simulink model "Copter_Plane_V10_sim_jy"  (R2021a)
settings: Solver=ode1  StartTime=0.0  StopTime=200  FixedStep=dt  RelTol=1e-3
undefined symbols (not defined in the file or in its folder): AC_Attitude, AC_PosControl, algo_accel_target_0, algo_accel_target_1, algo_accel_target_2, algo_arspeed, algo_attitude_target_euler_angle_0, algo_attitude_target_euler_angle_1, algo_attitude_target_euler_angle_2, algo_attitude_target_euler_rate_0, algo_attitude_target_euler_rate_1, algo_attitude_target_euler_rate_2, algo_climb_rate_cms, algo_curPathPoint_LLA_0, algo_curPathPoint_LLA_1, algo_curPosNED_0, algo_curPosNED_1, algo_curr_alt, algo_curr_pos_0, algo_curr_pos_1, algo_curr_vel_0, algo_curr_vel_1, algo_curr_vel_2, algo_current_loc_0, algo_current_loc_1, algo_curVelNED_0, algo_curVelNED_1, algo_flightControlMode, algo_flightTaskMode, algo_heightCmd_sl, algo_hgt_dem, algo_k_aileron, algo_k_elevator, algo_k_rudder, algo_k_throttle, algo_latAccDem, algo_limit_pos_up, algo_maxClimbSpeed, algo_mode, algo_nav_pitch_cd, algo_nav_roll, algo_pitch, algo_pitch_dem, algo_pitch_in, algo_pitch_target_pilot, algo_plane_mode, algo_pos_target_0, algo_pos_target_1, algo_pos_target_2, algo_prePathPoint_LLA_0, algo_prePathPoint_LLA_1, algo_pwm_out_1, algo_pwm_out_2, algo_pwm_out_3, algo_pwm_out_4, algo_rate_target_ang_vel_0, algo_rate_target_ang_vel_1, algo_rate_target_ang_vel_2, algo_remote_ct_st_pitch, algo_remote_ct_st_roll ... (+39)
libraries: aerolibasang x1, sharedtransform x1
(part 2 of 2)

== matlab function Copter_Plane_V10_sim_jy/input_euler_angle_roll_pitch_euler_rate_yaw ==
  data: GRAVITY_MSS data_store_memory; HD data_store_memory; dt data_store_memory; LOCATION_SCALING_FACTOR_INV data_store_memory; PathModeOut_sl data_store_memory; plane_mode data_store_memory; algo_remote_ct_st data_store_memory; algo_dbg_param data_store_memory; Curr_sate data_store_memory; systime data_store_memory; Test_w data_store_memory; AC_rate_pitch_pid data_store_memory; AC_rate_roll_pid data_store_memory; AC_rate_yaw_pid data_store_memory; AC_PosControl data_store_memory; AP_rate_roll data_store_memory; AP_rate_pitch data_store_memory; AP_rate_yaw data_store_memory; AP_TECS data_store_memory; AP_L1 data_store_memory; Plane data_store_memory; SRV_Channel data_store_memory; AC_Attitude data_store_memory; AP_Motors data_store_memory; Copter_Plane data_store_memory; LOCATION_SCALING_FACTOR data_store_memory; SINS data_store_memory; SlewLimiter data_store_memory
function copter_plane_run

run_remote();
load_Curr_sate();
loc_run();
load_inint();
sin_step_test();
%%%%%%%%%%%%%%%%%%%%%%%%%%%%
Copter_Plane_run();
%%%%%%%%%%%%%%%%%%%%%%%%%%%%
run_servo_pwm_adj();

end

== matlab function Copter_Plane_V10_sim_jy/MATLAB Function17 ==
  data: x_cmss input; forward output; y_cmss input; right output; SINS data_store_memory
function [forward, right]= to_body(  x_cmss,   y_cmss)  
global SINS
yaw =SINS.yaw;
    forward = x_cmss * cos(yaw) + y_cmss * sin(yaw);
    right = -x_cmss * sin(yaw) + y_cmss * cos(yaw);
